simulink model "LIDAR"  (R2023b)
settings: Solver=VariableStepAuto  StartTime=0.0  StopTime=10.0  RelTol=1e-3
settings Model: Creator=lucaerviati  LastModifiedBy=monis
settings OptimizationCC: ReuseModelBlockBuffer=off

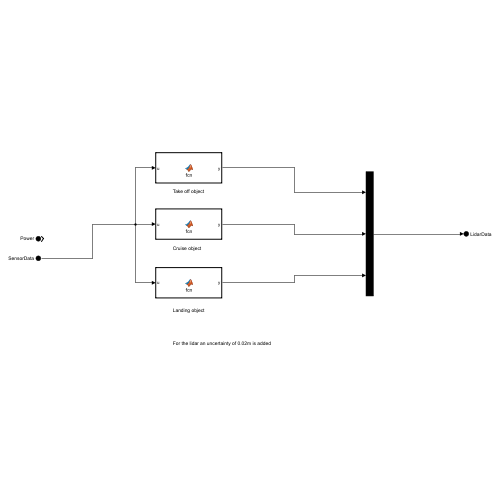
[thumbnail: Simulink's stored preview of the top-level diagram]
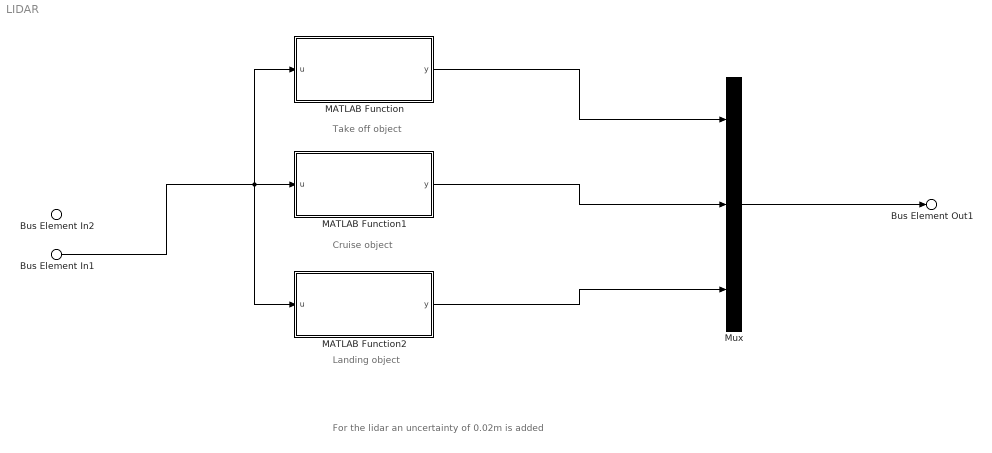
== system LIDAR ==
  note: For the lidar an uncertainty of 0.02m is added
  note: Cruise object
  note: Take off object
  note: Landing object
  Bus Element In2 : Inport  PortName=Power
  Bus Element In1 : Inport  Port=2  PortName=SensorData
  MATLAB Function : MATLAB Function  TreatAsAtomicUnit=on
  MATLAB Function1 : MATLAB Function  TreatAsAtomicUnit=on
  MATLAB Function2 : MATLAB Function  TreatAsAtomicUnit=on
  Mux : Mux  Inputs=3
  Bus Element Out1 : Outport  PortName=LidarData
  wires:
  Mux/1 -> Bus Element Out1/1
  MATLAB Function1/1(y) -> Mux/2
  Bus Element In1/1 -> MATLAB Function/1(u), MATLAB Function2/1(u), MATLAB Function1/1(u)
  MATLAB Function2/1(y) -> Mux/3
  MATLAB Function/1(y) -> Mux/1

== matlab function LIDAR/MATLAB Function ==
  data: u input; y output
function y = fcn(u)
u = [10,
    38,
    23]
y = u;

== matlab function LIDAR/MATLAB Function2 ==
  data: u input; y output
function y = fcn(u)
u = [22,
    33,
    66]
y = u;

== matlab function LIDAR/MATLAB Function1 ==
  data: u input; y output
function y = fcn(u)
u = [12,
    54,
    66]
y = u;
